simulink model "sl_computed_torque"  (R2022a)
settings: Solver=ode23t  StartTime=0.0  StopTime=5  FixedStep=0.01  MaxStep=0.05  RelTol=1e-3  EnableMultiTasking=on
PreLoadFcn:
  | if ~exist("ur5", "var")
  |    ur5 = loadrobot("universalUR5e", DataFormat="row", Gravity=[0 0 -9.81]);
  | end
  | 
  | if ~exist("ur5conf", "var")
  |   ur5conf.qn = [0 -1.07 1.38 -0.3 0 -2.3];
  |   ur5conf.qe = [0.9765 -0.8013 0.9933 -0.2655 0.8590 -2.2322];
  | end
InitFcn:
  | if ~exist("ur5", "var")
  |    ur5 = loadrobot("universalUR5e", DataFormat="row", Gravity=[0 0 -9.81]);
  | end
  | 
  | if ~exist("ur5conf", "var")
  |   ur5conf.qn = [0 -1.07 1.38 -0.3 0 -2.3];
  |   ur5conf.qe = [0.9765 -0.8013 0.9933 -0.2655 0.8590 -2.2322];
  | end
undefined symbols (not defined in the file or in its folder): qe2
libraries: robotmaniplib x2, robotcorelib x1
Description:
  | Computed torque control example for UR5 robot.
  | 
  | Robotics, Vision and Control - 3rd Edition; Section 9.4.2
settings Model: ExtModeTrigMode=oneshot  ExtModeArmWhenConnect=off  Creator=pic  LastModifiedBy=rpill
settings SolverCC: ZeroCrossControl=DisableAll  AlgebraicLoopSolver=TrustRegion  MaxZcPerStep=1
settings DataIOCC: SaveFormat=Array  SignalLoggingSaveFormat=ModelDataLogs  TimeSaveName=t  OutputSaveName=y  ReturnWorkspaceOutputsName=ctorque
settings OptimizationCC: BlockReduction=off  BooleanDataType=off  ExpressionDepthLimit=2147483647  InitFltsAndDblsToZero=on  LifeSpan=inf
settings DebuggingCC: SaveWithParameterizedLinksMsg=none  UnderspecifiedInitializationDetection=Classic  MergeDetectMultiDrivingBlocksExec=none  SignalResolutionControl=TryResolveAllWithWarning  MultiTaskDSMMsg=warning  MultiTaskCondExecSysMsg=none  FcnCallInpInsideContextMsg=warning  UnconnectedInputMsg=warning  UnconnectedOutputMsg=warning  UnconnectedLineMsg=warning  AllowSymbolicDim=off  StateNameClashWarn=warning  SFUnexpectedBacktrackingDiag=warning  SFNoUnconditionalDefaultTransitionDiag=warning  SFExecutionAtInitializationDiag=none  SFMachineParentedDataDiag=warning  ArithmeticOperatorsInVariantConditions=warning
settings HardwareCC: ProdBitPerPointer=32  ProdBitPerSizeT=32  ProdBitPerPtrDiffT=32  ProdLargestAtomicFloat=None  ProdIntDivRoundTo=Undefined  ProdEndianess=Unspecified  ProdWordSize=32  ProdHWDeviceType=32-bit Generic  TargetUnknown=on
settings ModelReferenceCC: PropagateSignalLabelsOutOfModel=off
settings SFSimCC: SimUseLocalCustomCode=off  CustomCodeUndefinedFunction=UseInterfaceOnly
settings RTWCC: RTWUseLocalCustomCode=off
settings CodeAppCC: StateflowObjectComments=on
settings GRTTargetCC: TargetLangStandard=C89/C90 (ANSI)  ModelReferenceCompliant=off  CompOptLevelCompliant=off  CombineOutputUpdateFcns=off  MatFileLogging=off  GRTInterface=on
settings ConfigComp: CovMetricSettings=dw  CovSaveCumulativeToWorkspaceVar=on  CovSaveSingleToWorkspaceVar=on  CovExternalEMLEnable=off

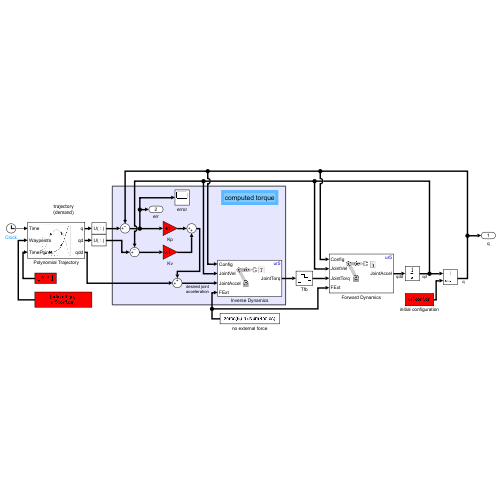
[thumbnail: Simulink's stored preview of the top-level diagram]
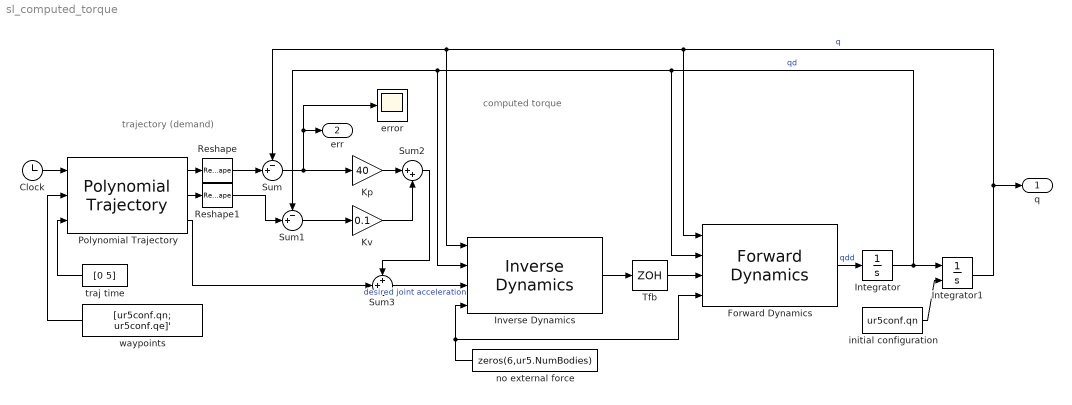
== system sl_computed_torque ==
  note: computed torque
  note: trajectory
      | (demand)
  Clock : Clock
  Forward Dynamics : robotmaniplib/Forward Dynamics  RigidBodyTree=ur5  SimulateUsing=Interpreted execution
  Integrator : Integrator
  Integrator1 : Integrator  InitialConditionSource=external
  Inverse Dynamics : robotmaniplib/Inverse Dynamics  RigidBodyTree=ur5  SimulateUsing=Interpreted execution
      settings: SourceProductBaseCode=RO
  Kp : Gain  Gain=40  SaturateOnIntegerOverflow=on  OutDataTypeStr=Inherit: Same as input  ParamDataTypeStr=Inherit: Same as input
  Kv : Gain  Gain=0.1  SaturateOnIntegerOverflow=on  OutDataTypeStr=Inherit: Same as input  ParamDataTypeStr=Inherit: Same as input
  Polynomial Trajectory : robotcorelib/Polynomial Trajectory  WaypointSource=External  Waypoints="[ur5conf.qn;  qe2]'"  TimePoints=[0, 5]  TimeInterval=[ 1, 4 ]  Method=Quintic Polynomial  ParameterSource=Internal  VelocityBoundaryCondition=zeros( 6, 2 )  AccelerationBoundaryCondition=zeros( 6, 2 )  SimulateUsing=Interpreted execution
      settings: SourceProductBaseCode=RO,NV,RR,UV
  Reshape : Reshape
  Reshape1 : Reshape
  Sum : Sum  Inputs=-+|  InputSameDT=on  SaturateOnIntegerOverflow=on  OutDataTypeStr=Inherit: Same as first input
  Sum1 : Sum  Inputs=-+|  InputSameDT=on  SaturateOnIntegerOverflow=on  OutDataTypeStr=Inherit: Same as first input
  Sum2 : Sum  Inputs=|++  InputSameDT=on  SaturateOnIntegerOverflow=on  OutDataTypeStr=Inherit: Same as first input
  Sum3 : Sum  Inputs=++|  InputSameDT=on  SaturateOnIntegerOverflow=on  OutDataTypeStr=Inherit: Same as first input
  Tfb : ZeroOrderHold  SampleTime=0.005
  error : Scope
  initial configuration : Constant  Value=ur5conf.qn
  no external force : Constant  Value=zeros(6,ur5.NumBodies)
  traj time : Constant  Value=[0 5]
  waypoints : Constant  Value=|
      | [ur5conf.qn; 
      | ur5conf.qe]'
  q : Outport  VectorParamsAs1DForOutWhenUnconnected=off
  err : Outport  Port=2  VectorParamsAs1DForOutWhenUnconnected=off
  wires:
  Sum/1 -> error/1, err/1, Kp/1
  Kp/1 -> Sum2/1
  Integrator1/1 -> q/1, Forward Dynamics/1, Inverse Dynamics/1, Sum/1  "q"
  Inverse Dynamics/1 -> Tfb/1
  Sum1/1 -> Kv/1
  Kv/1 -> Sum2/2
  Sum3/1 -> Inverse Dynamics/3  "desired joint acceleration"
  Tfb/1 -> Forward Dynamics/3
  Polynomial Trajectory/3 -> Sum3/2
  Sum2/1 -> Sum3/1
  initial configuration/1 -> Integrator1/2
  Forward Dynamics/1 -> Integrator/1  "qdd"
  Integrator/1 -> Sum1/1, Inverse Dynamics/2, Forward Dynamics/2, Integrator1/1  "qd"
  no external force/1 -> Forward Dynamics/4, Inverse Dynamics/4
  waypoints/1 -> Polynomial Trajectory/2
  Clock/1 -> Polynomial Trajectory/1
  traj time/1 -> Polynomial Trajectory/3
  Polynomial Trajectory/1 -> Reshape/1
  Reshape/1 -> Sum/2
  Polynomial Trajectory/2 -> Reshape1/1
  Reshape1/1 -> Sum1/2
